simulink model "main_system"  (R2025b)
settings: Solver=ode45  StartTime=0.0  StopTime=0.4  FixedStep=1e-05  MaxStep=1e-06  RelTol=1e-3
undefined symbols (not defined in the file or in its folder): alloc_params, ControllerType, delay_steps, model_base_ctrl_params, motion_control_law_params, p0, particle_dynamics_params, pi_ctrl_params, signal_type, thermal_force_params, trajectory_generator_params, vd_signal_params
libraries: simulink x1
settings Model: Creator=PME406_01  LastModifiedBy=kevin
settings DebuggingCC: MergeDetectMultiDrivingBlocksExec=none
settings ModelReferenceCC: PropagateSignalLabelsOutOfModel=off

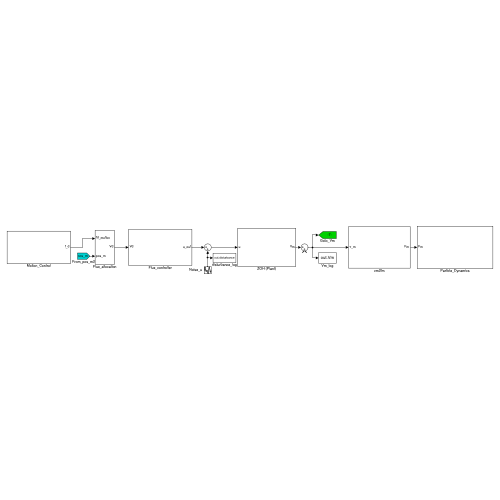
[thumbnail: Simulink's stored preview of the top-level diagram]
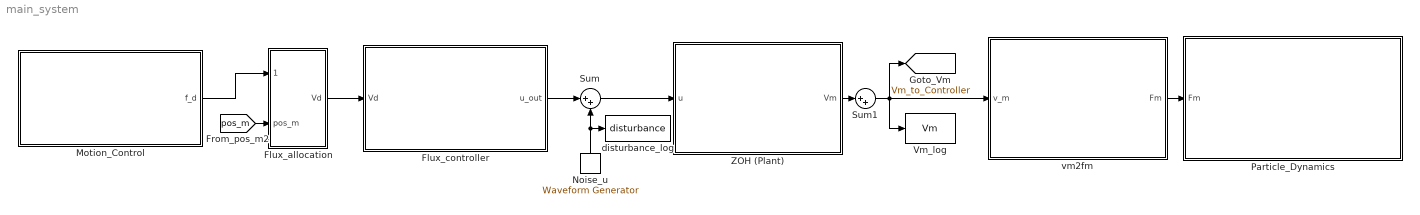
== system main_system ==
  Flux_allocation : Subsystem
  Flux_controller : Subsystem
  Motion_Control : Subsystem
  Noise_u : simulink/Sources/Waveform Generator  OutMin=[]  OutMax=[]  OutDataTypeStr=double  SelectedSignal=7  Signals=sin(0.1,10*2*pi, 0) + sin(0.1, 100*2*pi, pi/2) +sin(0.1,1000*2*pi, pi/4)#square(0.1,1000*2*pi,0,50)+square(0.1,500*2*pi,0,50)+square(0.1,50*2*pi,0,50)#sin(0.1,100*2*pi, pi/4)+sin(0.1,3000*2*pi,0)#square(0.1,50*2*pi,0,50)#sin(0.3, 100*2*pi, 0)#sawtooth(0.15,100*2*pi, pi/2)+sin(0.3, 100*2*pi, 0)#  BlockNames=MultiportSwitch_6f71199b286f490#MultiportSwitch_dade89289388493#MultiportSwitch_cf8a6d85c6a04a6#MultiportSwitch_8069dea399c144f#MultiportSwitch_735d7398da51477#MultiportSwitch_ae675588fc81459#MultiportSwitch_89d8400a71a24e9  SampleTime=1e-5
  Particle_Dynamics : Subsystem
  Sum : Sum  Inputs=|++
  Sum1 : Sum  Inputs=|++
  Vm_log : ToWorkspace  VariableName=Vm  SampleTime=1e-5
      settings: Save2DSignal=2-D array (concatenate along first dimension)
  ZOH (Plant) : Subsystem
  disturbance_log : ToWorkspace  VariableName=disturbance  SampleTime=1e-5
      settings: Save2DSignal=2-D array (concatenate along first dimension)
  vm2fm : Subsystem
  tag scope: Vm_to_Controller=global
  wires:
  Noise_u/1 -> disturbance_log/1, Sum/2
  Sum/1 -> ZOH (Plant)/1(u)
  ZOH (Plant)/1(Vm) -> Sum1/1
  Flux_controller/1(u_out) -> Sum/1
  Flux_allocation/1(Vd) -> Flux_controller/1(Vd)
  vm2fm/1(Fm) -> Particle_Dynamics/1(Fm)
  Motion_Control/1(f_d) -> Flux_allocation/1(fd_motion)
  Sum1/1 -> vm2fm/1(v_m), [Vm_to_Controller], Vm_log/1
  [pos_m] -> Flux_allocation/2(pos_m)

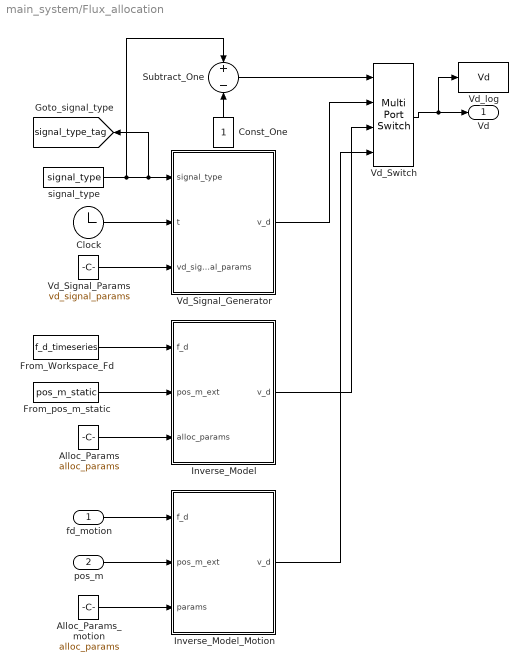
== system main_system/Flux_allocation ==
  fd_motion : Inport
  pos_m : Inport  Port=2
  Alloc_Params : Constant  Value=alloc_params  OutDataTypeStr=Bus: ForceModelAllocationParamsBus
  Alloc_Params_motion : Constant  Value=alloc_params  OutDataTypeStr=Bus: ForceModelAllocationParamsBus
  Clock : Clock
  Const_One : Constant
  From_Workspace_Fd : FromWorkspace  VariableName=f_d_timeseries  SampleTime=1e-5  OutputAfterFinalValue=Holding final value
  From_pos_m_static : FromWorkspace  VariableName=pos_m_static
  Inverse_Model : MATLAB Function  TreatAsAtomicUnit=on
  Inverse_Model_Motion : MATLAB Function  TreatAsAtomicUnit=on
  Subtract_One : Sum  Inputs=+-
  Vd_Signal_Generator : MATLAB Function  TreatAsAtomicUnit=on
  Vd_Signal_Params : Constant  Value=vd_signal_params  OutDataTypeStr=Bus: VdSignalParamsBus
  Vd_Switch : MultiPortSwitch  DataPortOrder=Zero-based contiguous  zeroidx=on  SaturateOnIntegerOverflow=off  InputSameDT=off
  Vd_log : ToWorkspace  VariableName=Vd  SampleTime=1e-5
      settings: Save2DSignal=2-D array (concatenate along first dimension)
  signal_type : Constant  Value=signal_type
  Vd : Outport
  tag scope: signal_type_tag=global
  wires:
  Clock/1 -> Vd_Signal_Generator/2(t)
  Subtract_One/1 -> Vd_Switch/1
  signal_type/1 -> [signal_type_tag], Vd_Signal_Generator/1(signal_type), Subtract_One/1
  Const_One/1 -> Subtract_One/2
  Vd_Switch/1 -> Vd/1, Vd_log/1
  Vd_Signal_Params/1 -> Vd_Signal_Generator/3(vd_signal_params)
  Alloc_Params/1 -> Inverse_Model/3(alloc_params)
  From_Workspace_Fd/1 -> Inverse_Model/1(f_d)
  Vd_Signal_Generator/1(v_d) -> Vd_Switch/2
  Inverse_Model/1(v_d) -> Vd_Switch/3
  Alloc_Params_motion/1 -> Inverse_Model_Motion/3(params)
  Inverse_Model_Motion/1(v_d) -> Vd_Switch/4
  fd_motion/1 -> Inverse_Model_Motion/1(f_d)
  pos_m/1 -> Inverse_Model_Motion/2(pos_m_ext)
  From_pos_m_static/1 -> Inverse_Model/2(pos_m_ext)

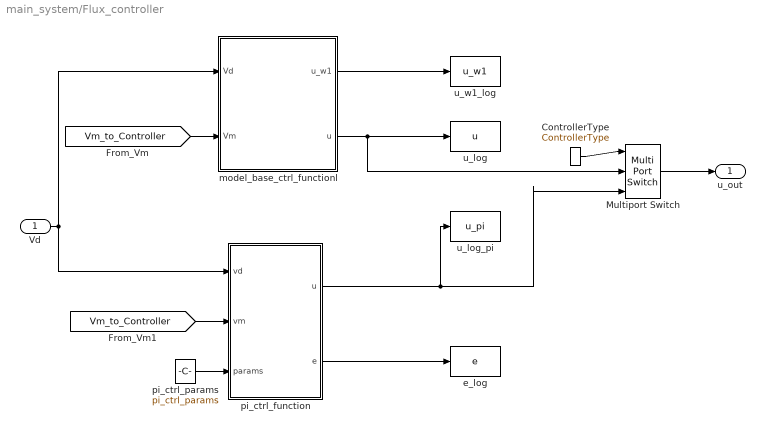
== system main_system/Flux_controller ==
  Vd : Inport
  ControllerType : Constant  Value=ControllerType
  Multiport Switch : MultiPortSwitch  Inputs=2  SaturateOnIntegerOverflow=off  InputSameDT=off
  e_log : ToWorkspace  VariableName=e  SampleTime=1e-5
      settings: Save2DSignal=2-D array (concatenate along first dimension)
  model_base_ctrl_functionl : Subsystem
  pi_ctrl_function : MATLAB Function  TreatAsAtomicUnit=on
  pi_ctrl_params : Constant  Value=pi_ctrl_params  OutDataTypeStr=Bus: PICtrlParamsBus
  u_log : ToWorkspace  VariableName=u  SampleTime=1e-5
      settings: Save2DSignal=2-D array (concatenate along first dimension)
  u_log_pi : ToWorkspace  VariableName=u_pi  SampleTime=1e-5
      settings: Save2DSignal=2-D array (concatenate along first dimension)
  u_w1_log : ToWorkspace  VariableName=u_w1  SampleTime=1e-5
      settings: Save2DSignal=2-D array (concatenate along first dimension)
  u_out : Outport
  wires:
  Vd/1 -> pi_ctrl_function/1(vd), model_base_ctrl_functionl/1(Vd)
  pi_ctrl_function/1(u) -> u_log_pi/1, Multiport Switch/3
  ControllerType/1 -> Multiport Switch/1
  [Vm_to_Controller] -> pi_ctrl_function/2(vm)
  model_base_ctrl_functionl/1(u_w1) -> u_w1_log/1
  model_base_ctrl_functionl/2(u) -> u_log/1, Multiport Switch/2
  [Vm_to_Controller] -> model_base_ctrl_functionl/2(Vm)
  Multiport Switch/1 -> u_out/1
  pi_ctrl_function/2(e) -> e_log/1
  pi_ctrl_params/1 -> pi_ctrl_function/3(params)

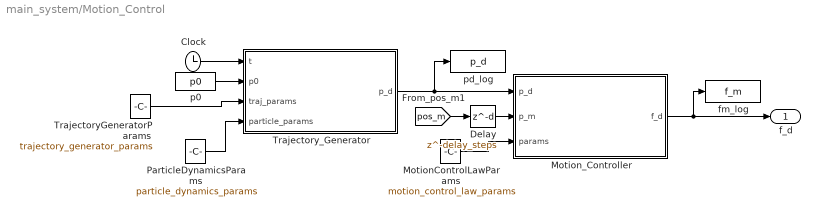
== system main_system/Motion_Control ==
  Clock : Clock
  Delay : Delay  DelayLength=delay_steps  InitialCondition=repmat(p0, 1, max(1, delay_steps))  SampleTime=1/1600
  MotionControlLawParams : Constant  Value=motion_control_law_params  OutDataTypeStr=Bus: MotionControlLawParamsBus
  Motion_Controller : MATLAB Function  TreatAsAtomicUnit=on
  ParticleDynamicsParams : Constant  Value=particle_dynamics_params  OutDataTypeStr=Bus: ParticleDynamicsParamsBus
  TrajectoryGeneratorParams : Constant  Value=trajectory_generator_params  OutDataTypeStr=Bus: TrajectoryGeneratorParamsBus
  Trajectory_Generator : MATLAB Function  TreatAsAtomicUnit=on
  fm_log : ToWorkspace  VariableName=f_m  SampleTime=1e-5
      settings: Save2DSignal=2-D array (concatenate along first dimension)
  p0 : Constant  Value=p0
  pd_log : ToWorkspace  VariableName=p_d  SampleTime=1e-5
      settings: Save2DSignal=2-D array (concatenate along first dimension)
  f_d : Outport
  wires:
  p0/1 -> Trajectory_Generator/2(p0)
  Clock/1 -> Trajectory_Generator/1(t)
  TrajectoryGeneratorParams/1 -> Trajectory_Generator/3(traj_params)
  Trajectory_Generator/1(p_d) -> pd_log/1, Motion_Controller/1(p_d)
  Motion_Controller/1(f_d) -> fm_log/1, f_d/1
  MotionControlLawParams/1 -> Motion_Controller/3(params)
  ParticleDynamicsParams/1 -> Trajectory_Generator/4(particle_params)
  [pos_m] -> Delay/1
  Delay/1 -> Motion_Controller/2(p_m)

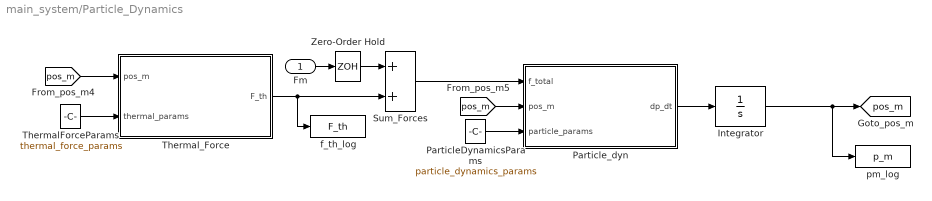
== system main_system/Particle_Dynamics ==
  Fm : Inport
  Integrator : Integrator  InitialCondition=p0
  ParticleDynamicsParams : Constant  Value=particle_dynamics_params  OutDataTypeStr=Bus: ParticleDynamicsParamsBus
  Particle_dyn : MATLAB Function  TreatAsAtomicUnit=on
  Sum_Forces : Sum
  ThermalForceParams : Constant  Value=thermal_force_params  OutDataTypeStr=Bus: ThermalForceParamsBus
  Thermal_Force : MATLAB Function  TreatAsAtomicUnit=on
  Zero-Order Hold : ZeroOrderHold  SampleTime=1/1600
  f_th_log : ToWorkspace  VariableName=F_th  SampleTime=1e-5
      settings: Save2DSignal=2-D array (concatenate along first dimension)
  pm_log : ToWorkspace  VariableName=p_m  SampleTime=1e-5
      settings: Save2DSignal=2-D array (concatenate along first dimension)
  tag scope: pos_m=global
  wires:
  ParticleDynamicsParams/1 -> Particle_dyn/3(particle_params)
  ThermalForceParams/1 -> Thermal_Force/2(thermal_params)
  Thermal_Force/1(F_th) -> f_th_log/1, Sum_Forces/2
  Sum_Forces/1 -> Particle_dyn/1(f_total)
  Particle_dyn/1(dp_dt) -> Integrator/1
  Fm/1 -> Zero-Order Hold/1
  Zero-Order Hold/1 -> Sum_Forces/1
  [pos_m] -> Particle_dyn/2(pos_m)
  [pos_m] -> Thermal_Force/1(pos_m)
  Integrator/1 -> pm_log/1, [pos_m]

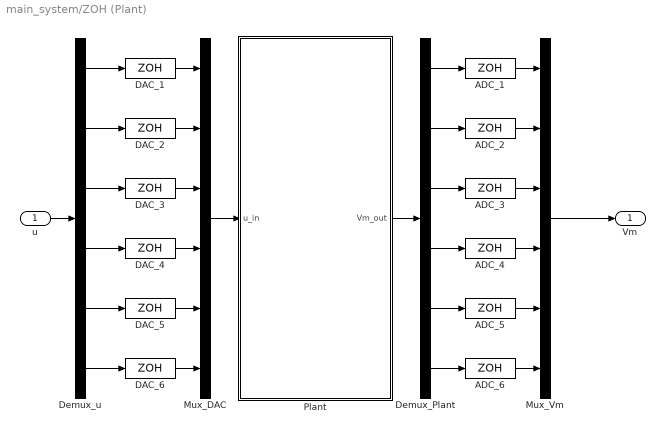
== system main_system/ZOH (Plant) ==
  u : Inport
  ADC_{1..6} (6 alike) : ZeroOrderHold  SampleTime=1e-05
  DAC_{1..6} (6 alike) : ZeroOrderHold  SampleTime=1e-05
  Demux_Plant : Demux  Outputs=6
  Demux_u : Demux  Outputs=6
  Mux_DAC : Mux  Inputs=6
  Mux_Vm : Mux  Inputs=6
  Plant : Subsystem
  Vm : Outport
  wires:
  Demux_Plant/3 -> ADC_3/1
  DAC_2/1 -> Mux_DAC/2
  Demux_u/1 -> DAC_1/1
  Demux_u/6 -> DAC_6/1
  ADC_4/1 -> Mux_Vm/4
  DAC_3/1 -> Mux_DAC/3
  Mux_Vm/1 -> Vm/1
  Demux_Plant/2 -> ADC_2/1
  ADC_6/1 -> Mux_Vm/6
  Demux_Plant/1 -> ADC_1/1
  ADC_2/1 -> Mux_Vm/2
  Demux_u/5 -> DAC_5/1
  Plant/1(Vm_out) -> Demux_Plant/1
  Mux_DAC/1 -> Plant/1(u_in)
  DAC_1/1 -> Mux_DAC/1
  ADC_1/1 -> Mux_Vm/1
  Demux_u/4 -> DAC_4/1
  Demux_u/3 -> DAC_3/1
  Demux_Plant/6 -> ADC_6/1
  Demux_Plant/4 -> ADC_4/1
  ADC_3/1 -> Mux_Vm/3
  Demux_Plant/5 -> ADC_5/1
  DAC_4/1 -> Mux_DAC/4
  ADC_5/1 -> Mux_Vm/5
  DAC_5/1 -> Mux_DAC/5
  DAC_6/1 -> Mux_DAC/6
  Demux_u/2 -> DAC_2/1
  u/1 -> Demux_u/1

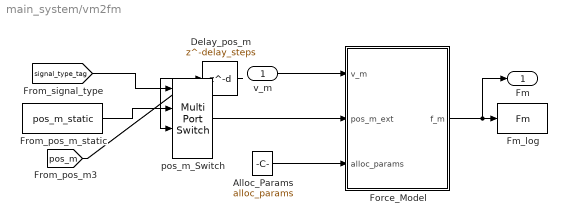
== system main_system/vm2fm ==
  v_m : Inport
  Alloc_Params : Constant  Value=alloc_params  OutDataTypeStr=Bus: ForceModelAllocationParamsBus
  Delay_pos_m : Delay  DelayLength=delay_steps  InitialCondition=repmat(p0, 1, max(1, delay_steps))  SampleTime=1/1600
  Fm_log : ToWorkspace  VariableName=Fm  SaveFormat=Timeseries  SampleTime=1e-5
      settings: Save2DSignal=2-D array (concatenate along first dimension)
  Force_Model : MATLAB Function  TreatAsAtomicUnit=on
  From_pos_m_static : FromWorkspace  VariableName=pos_m_static
  pos_m_Switch : MultiPortSwitch  SaturateOnIntegerOverflow=off  InputSameDT=off
  Fm : Outport
  wires:
  v_m/1 -> Force_Model/1(v_m)
  Alloc_Params/1 -> Force_Model/3(alloc_params)
  Force_Model/1(f_m) -> Fm/1, Fm_log/1
  pos_m_Switch/1 -> Force_Model/2(pos_m_ext)
  [signal_type_tag] -> pos_m_Switch/1
  From_pos_m_static/1 -> pos_m_Switch/2
  [pos_m] -> Delay_pos_m/1
  Delay_pos_m/1 -> pos_m_Switch/3

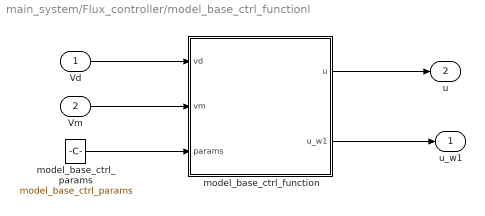
== system main_system/Flux_controller/model_base_ctrl_functionl ==
  Vd : Inport
  Vm : Inport  Port=2
  model_base_ctrl_function : MATLAB Function  TreatAsAtomicUnit=on
  model_base_ctrl_params : Constant  Value=model_base_ctrl_params  OutDataTypeStr=Bus: ModelBaseCtrlParamsBus
  u_w1 : Outport
  u : Outport  Port=2
  wires:
  model_base_ctrl_function/2(u_w1) -> u_w1/1
  Vm/1 -> model_base_ctrl_function/2(vm)
  Vd/1 -> model_base_ctrl_function/1(vd)
  model_base_ctrl_function/1(u) -> u/1
  model_base_ctrl_params/1 -> model_base_ctrl_function/3(params)

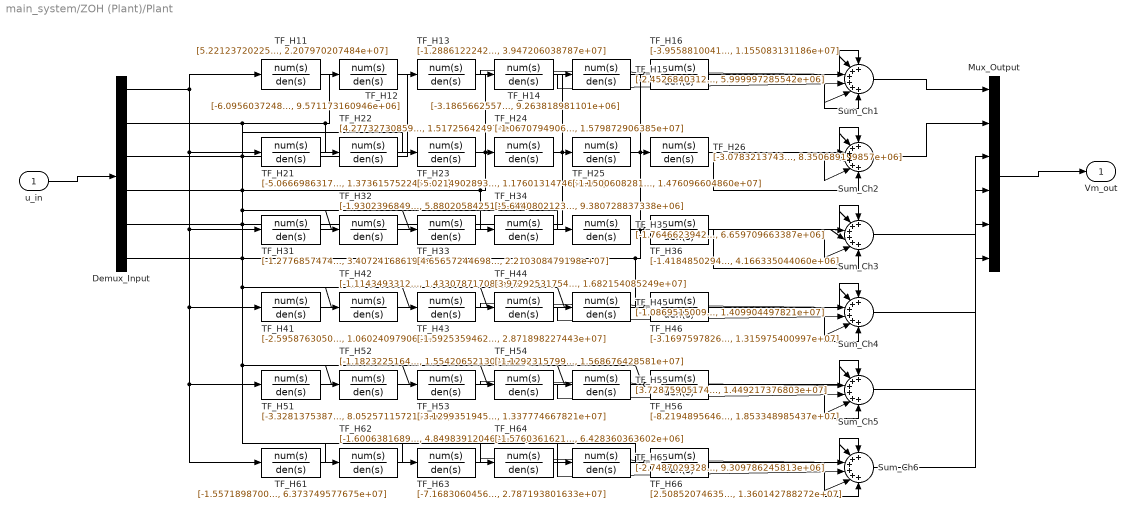
== system main_system/ZOH (Plant)/Plant ==
  u_in : Inport
  Demux_Input : Demux  Outputs=6
  Mux_Output : Mux  Inputs=6
  Sum_Ch{1..6} (6 alike) : Sum  Inputs=++++++
  TF_H11 : TransferFcn  Numerator=[5.221237202258e+06]  Denominator=[1, 1.125476429798e+04, 2.207970207484e+07]
  TF_H12 : TransferFcn  Numerator=[-6.095603724823e+04]  Denominator=[1, 1.615096196557e+03, 9.571173160946e+06]
  TF_H13 : TransferFcn  Numerator=[-1.288612224236e+06]  Denominator=[1, 1.231137597589e+04, 3.947206038787e+07]
  TF_H14 : TransferFcn  Numerator=[-3.186566255776e+05]  Denominator=[1, 7.765927137710e+03, 9.263818981101e+06]
  TF_H15 : TransferFcn  Numerator=[-2.452684031253e+05]  Denominator=[1, 5.746401647961e+03, 5.999997285542e+06]
  TF_H16 : TransferFcn  Numerator=[-3.955881004140e+05]  Denominator=[1, 3.580306515557e+03, 1.155083131186e+07]
  TF_H21 : TransferFcn  Numerator=[-5.066698631790e+04]  Denominator=[1, 1.108261849372e+03, 1.373615752245e+07]
  TF_H22 : TransferFcn  Numerator=[4.277327308593e+06]  Denominator=[1, 1.003268373777e+04, 1.517256424974e+07]
  TF_H23 : TransferFcn  Numerator=[-5.021490289304e+05]  Denominator=[1, 8.810895080316e+03, 1.176013147465e+07]
  TF_H24 : TransferFcn  Numerator=[-1.067079490600e+06]  Denominator=[1, 1.135112820448e+04, 1.579872906385e+07]
  TF_H25 : TransferFcn  Numerator=[-1.150060828107e+06]  Denominator=[1, 1.065992916636e+04, 1.476096604860e+07]
  TF_H26 : TransferFcn  Numerator=[-3.078321374306e+05]  Denominator=[1, 6.847783968129e+03, 8.350689199857e+06]
  TF_H31 : TransferFcn  Numerator=[-1.277685747428e+06]  Denominator=[1, 1.368269686933e+04, 3.407241686199e+07]
  TF_H32 : TransferFcn  Numerator=[-1.930239684968e+05]  Denominator=[1, 4.560870597302e+03, 5.880205842512e+06]
  TF_H33 : TransferFcn  Numerator=[4.656572446985e+06]  Denominator=[1, 9.513164457161e+03, 2.210308479198e+07]
  TF_H34 : TransferFcn  Numerator=[-5.644080212304e+04]  Denominator=[1, 1.954878812118e+03, 9.380728837338e+06]
  TF_H35 : TransferFcn  Numerator=[-1.764662394212e+05]  Denominator=[1, 5.122349981324e+03, 6.659709663387e+06]
  TF_H36 : TransferFcn  Numerator=[-1.418485029440e+05]  Denominator=[1, 1.438504147902e+03, 4.166335044060e+06]
  TF_H41 : TransferFcn  Numerator=[-2.595876305066e+05]  Denominator=[1, 7.070165651413e+03, 1.060240979066e+07]
  TF_H42 : TransferFcn  Numerator=[-1.114349331223e+06]  Denominator=[1, 9.846928206402e+03, 1.433078717084e+07]
  TF_H43 : TransferFcn  Numerator=[-1.592535946272e+05]  Denominator=[1, 2.790294019501e+03, 2.871898227443e+07]
  TF_H44 : TransferFcn  Numerator=[3.972925317547e+06]  Denominator=[1, 1.159715140811e+04, 1.682154085249e+07]
  TF_H45 : TransferFcn  Numerator=[-1.086951500933e+06]  Denominator=[1, 1.075231371220e+04, 1.409904497821e+07]
  TF_H46 : TransferFcn  Numerator=[-3.169759782656e+05]  Denominator=[1, 8.067558736035e+03, 1.315975400997e+07]
  TF_H51 : TransferFcn  Numerator=[-3.328137538766e+05]  Denominator=[1, 7.227274813518e+03, 8.052571157216e+06]
  TF_H52 : TransferFcn  Numerator=[-1.182322516481e+06]  Denominator=[1, 1.030784744910e+04, 1.554206521303e+07]
  TF_H53 : TransferFcn  Numerator=[-3.129935194599e+05]  Denominator=[1, 7.870328655037e+03, 1.337774667821e+07]
  TF_H54 : TransferFcn  Numerator=[-1.129231579925e+06]  Denominator=[1, 1.104821595243e+04, 1.568676428581e+07]
  TF_H55 : TransferFcn  Numerator=[3.728759051745e+06]  Denominator=[1, 1.050075182774e+04, 1.449217376803e+07]
  TF_H56 : TransferFcn  Numerator=[-8.219489564647e+04]  Denominator=[1, 1.407969854523e+03, 1.853348985437e+07]
  TF_H61 : TransferFcn  Numerator=[-1.557189870041e+06]  Denominator=[1, 2.234640585923e+04, 6.373749577675e+07]
  TF_H62 : TransferFcn  Numerator=[-1.600638168987e+05]  Denominator=[1, 3.864055922471e+03, 4.849839120469e+06]
  TF_H63 : TransferFcn  Numerator=[-7.168306045699e+05]  Denominator=[1, 9.251556589809e+03, 2.787193801633e+07]
  TF_H64 : TransferFcn  Numerator=[-1.576036162155e+05]  Denominator=[1, 4.743270970318e+03, 6.428360363602e+06]
  TF_H65 : TransferFcn  Numerator=[-2.748702932822e+04]  Denominator=[1, 4.876033357949e+02, 9.309786245813e+06]
  TF_H66 : TransferFcn  Numerator=[2.508520746356e+06]  Denominator=[1, 5.985310903650e+03, 1.360142788272e+07]
  Vm_out : Outport
  wires:
  Sum_Ch3/1 -> Mux_Output/3
  TF_H36/1 -> Sum_Ch3/6
  TF_H16/1 -> Sum_Ch1/6
  TF_H63/1 -> Sum_Ch6/3
  Demux_Input/2 -> TF_H52/1, TF_H62/1, TF_H42/1, TF_H32/1, TF_H12/1, TF_H22/1
  TF_H23/1 -> Sum_Ch2/3
  TF_H31/1 -> Sum_Ch3/1
  Sum_Ch1/1 -> Mux_Output/1
  TF_H51/1 -> Sum_Ch5/1
  TF_H12/1 -> Sum_Ch1/2
  TF_H61/1 -> Sum_Ch6/1
  TF_H22/1 -> Sum_Ch2/2
  Demux_Input/4 -> TF_H54/1, TF_H64/1, TF_H44/1, TF_H14/1, TF_H24/1, TF_H34/1
  TF_H14/1 -> Sum_Ch1/4
  TF_H62/1 -> Sum_Ch6/2
  TF_H25/1 -> Sum_Ch2/5
  Sum_Ch4/1 -> Mux_Output/4
  TF_H41/1 -> Sum_Ch4/1
  TF_H45/1 -> Sum_Ch4/5
  Sum_Ch6/1 -> Mux_Output/6
  TF_H54/1 -> Sum_Ch5/4
  TF_H64/1 -> Sum_Ch6/4
  TF_H55/1 -> Sum_Ch5/5
  Demux_Input/6 -> TF_H56/1, TF_H66/1, TF_H16/1, TF_H26/1, TF_H36/1, TF_H46/1
  TF_H42/1 -> Sum_Ch4/2
  TF_H13/1 -> Sum_Ch1/3
  TF_H26/1 -> Sum_Ch2/6
  TF_H21/1 -> Sum_Ch2/1
  Demux_Input/5 -> TF_H55/1, TF_H65/1, TF_H45/1, TF_H15/1, TF_H25/1, TF_H35/1
  Sum_Ch2/1 -> Mux_Output/2
  u_in/1 -> Demux_Input/1
  TF_H44/1 -> Sum_Ch4/4
  TF_H24/1 -> Sum_Ch2/4
  TF_H66/1 -> Sum_Ch6/6
  TF_H43/1 -> Sum_Ch4/3
  TF_H33/1 -> Sum_Ch3/3
  TF_H52/1 -> Sum_Ch5/2
  Demux_Input/3 -> TF_H53/1, TF_H63/1, TF_H43/1, TF_H33/1, TF_H13/1, TF_H23/1
  TF_H15/1 -> Sum_Ch1/5
  TF_H56/1 -> Sum_Ch5/6
  TF_H32/1 -> Sum_Ch3/2
  TF_H34/1 -> Sum_Ch3/4
  TF_H53/1 -> Sum_Ch5/3
  Demux_Input/1 -> TF_H51/1, TF_H61/1, TF_H41/1, TF_H31/1, TF_H21/1, TF_H11/1
  TF_H11/1 -> Sum_Ch1/1
  TF_H35/1 -> Sum_Ch3/5
  Mux_Output/1 -> Vm_out/1
  Sum_Ch5/1 -> Mux_Output/5
  TF_H65/1 -> Sum_Ch6/5
  TF_H46/1 -> Sum_Ch4/6

== matlab function main_system/Flux_controller/model_base_ctrl_functionl/model_base_ctrl_function ==
  settings: updateMethod=DISCRETE  sampleTime=1e-5
  data: vd input size=6; u output size=6; vm input size=6; u_w1 output size=6; params input
function [u, u_w1] = fcn(vd, vm, params)
    [u, u_w1] = model_base_ctrl_function(vd, vm, params);
end

== matlab function main_system/Flux_allocation/Vd_Signal_Generator ==
  settings: updateMethod=DISCRETE  sampleTime=1e-5
  data: signal_type input; t input; vd_signal_params input; v_d output size=6
 function v_d = Vd_Signal_Generator(signal_type, t, vd_signal_params)
      v_d = vd_signal_function(signal_type, t, vd_signal_params);
 end

== matlab function main_system/Flux_controller/pi_ctrl_function ==
  settings: updateMethod=DISCRETE  sampleTime=1e-5
  data: vd input size=6; u output size=6; vm input size=6; params input; e output size=6
function [u, e] = fcn(vd, vm, params)
      [u, e] = pi_ctrl_function(vd, vm, params);
end

== matlab function main_system/Flux_allocation/Inverse_Model ==
  settings: updateMethod=DISCRETE  sampleTime=1e-5
  data: f_d input size=3; pos_m_ext input; alloc_params input; v_d output size=6
function v_d = Inverse_Model(f_d, pos_m_ext, alloc_params)
      v_d = inverse_model_function(f_d, pos_m_ext, alloc_params);
end

== matlab function main_system/vm2fm/Force_Model ==
  settings: updateMethod=DISCRETE  sampleTime=1e-5
  data: v_m input size=6; pos_m_ext input; alloc_params input; f_m output size=3
function f_m = Force_Model(v_m, pos_m_ext, alloc_params)
      f_m = force_model_function(v_m, pos_m_ext, alloc_params);
end

== matlab function main_system/Flux_allocation/Inverse_Model_Motion ==
  settings: updateMethod=DISCRETE  sampleTime=1e-5
  data: f_d input size=3; pos_m_ext input size=3; v_d output size=6; params input
function v_d = fcn(f_d, pos_m_ext, params)
      v_d = inverse_model_function(f_d, pos_m_ext, params);
end

== matlab function main_system/Motion_Control/Motion_Controller ==
  settings: updateMethod=DISCRETE  sampleTime=1/1600
  data: p_d input size=3; f_d output size=3; p_m input size=3; params input
function f_d = fcn(p_d, p_m, params)
    f_d = motion_control_law_function(p_d, p_m, params);
end

== matlab function main_system/Motion_Control/Trajectory_Generator ==
  settings: updateMethod=DISCRETE  sampleTime=1/1600
  data: t input; p_d output size=3; p0 input size=3; traj_params input Bus: TrajectoryGeneratorParamsBus; particle_params input Bus: ParticleDynamicsParamsBus
function p_d = fcn(t, p0, traj_params, particle_params)
%#codegen

    % Initialize output
    p_d = p0;

    if traj_params.type < 0.5  % z_sine
        % Wall normal direction
        w_hat = particle_params.w_hat;
        amplitude = traj_params.amplitude;
        frequency = traj_params.frequency;
        n_cycles = traj_params.n_cycles;
        T_total = n_cycles / frequency;

        if t <= T_total
            omega = 2 * pi * frequency;
            displacement = amplitude * sin(omega * t);
            p_d = p0 + displacement * w_hat;
        end

    elseif traj_params.type < 1.5  % xy_circle
        x_hat = [1; 0; 0];
        y_hat = [0; 1; 0];
        radius = traj_params.radius;
        period = traj_params.period;
        n_cycles = traj_params.n_cycles;
        T_total = period * n_cycles;

        if t <= T_total
            omega = 2 * pi / period;
            p_d = p0 + radius * (cos(omega * t) - 1) * x_hat ...
                     + radius * sin(omega * t) * y_hat;
        end

    end
    % positioning (type >= 1.5): p_d = p0 (already initialized)

end

== matlab function main_system/Particle_Dynamics/Thermal_Force ==
  settings: updateMethod=DISCRETE  sampleTime=1/1600
  data: pos_m input size=3; F_th output size=3; thermal_params input Bus: ThermalForceParamsBus
function F_th = Thermal_Force(pos_m, thermal_params)
      F_th = calc_thermal_force_function(pos_m, thermal_params);
end

== matlab function main_system/Particle_Dynamics/Particle_dyn ==
  settings: updateMethod=DISCRETE  sampleTime=1/1600
  data: f_total input size=3; pos_m input size=3; dp_dt output size=3; particle_params input Bus: ParticleDynamicsParamsBus
function dp_dt = Particle_ODE(f_total, pos_m, particle_params)
      if particle_params.wall_effect_enable > 0.5
          [Gamma_inv, ~] = calc_gamma_inv_function(pos_m, particle_params);
      else
          Gamma_inv = eye(3) / particle_params.gamma_N;
      end
      dp_dt = Gamma_inv * f_total;
end
